simulink model "LAB4_secondoEs"  (R2025b)
settings: Solver=ode45  StartTime=0.0  StopTime=Tend  MaxStep=0.001*Ts  MinStep=0.0001*Ts  RelTol=1e-3
undefined symbols (not defined in the file): C, DiscIntNeverNeededParam, K_q, K_x, step_value, Ts, x0i
libraries: cstblocks x1
settings Model: Creator=davidecovolo  LastModifiedBy=davidecovolo
settings SolverCC: InitialStep=0.0001*Ts

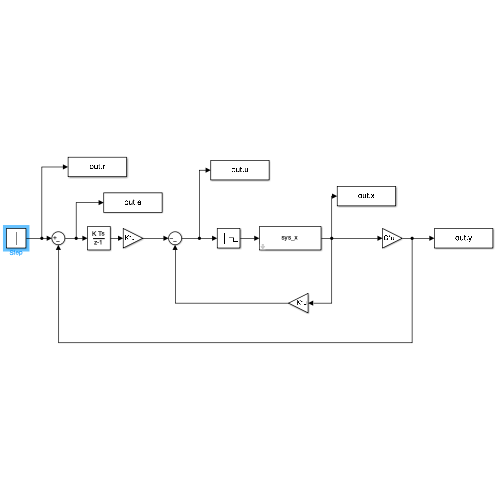
[thumbnail: Simulink's stored preview of the top-level diagram]
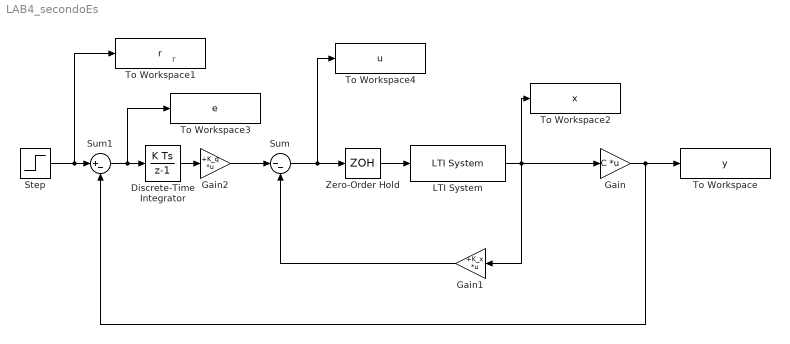
== system LAB4_secondoEs ==
  note: r
  Discrete-Time Integrator : DiscreteIntegrator  InitialCondition=x0i  SampleTime=Ts  ICPrevOutput=DiscIntNeverNeededParam  ICPrevScaledInput=DiscIntNeverNeededParam
  Gain : Gain  Gain=C  Multiplication=Matrix(K*u)
  Gain1 : Gain  Gain=+K_x  Multiplication=Matrix(K*u)
  Gain2 : Gain  Gain=+K_q  Multiplication=Matrix(K*u)
  LTI System : cstblocks/LTI System  sys=sys_x  IC=x0  PadeOrder=0
  Step : Step  Time=0  After=step_value  SampleTime=Ts
  Sum : Sum  Inputs=|--
  Sum1 : Sum  Inputs=|+-
  To Workspace : ToWorkspace  VariableName=y  SaveFormat=Timeseries  SampleTime=Ts
  To Workspace1 : ToWorkspace  VariableName=r  SaveFormat=Timeseries  SampleTime=Ts
  To Workspace2 : ToWorkspace  VariableName=x  SaveFormat=Timeseries  SampleTime=Ts
  To Workspace3 : ToWorkspace  VariableName=e  SaveFormat=Timeseries  SampleTime=Ts
  To Workspace4 : ToWorkspace  VariableName=u  SaveFormat=Timeseries  SampleTime=Ts
  Zero-Order Hold : ZeroOrderHold  SampleTime=Ts
  wires:
  Gain1/1 -> Sum/2
  LTI System/1 -> To Workspace2/1, Gain/1, Gain1/1
  Zero-Order Hold/1 -> LTI System/1
  Sum/1 -> To Workspace4/1, Zero-Order Hold/1
  Gain2/1 -> Sum/1
  Discrete-Time Integrator/1 -> Gain2/1
  Step/1 -> To Workspace1/1, Sum1/1
  Gain/1 -> Sum1/2, To Workspace/1
  Sum1/1 -> To Workspace3/1, Discrete-Time Integrator/1
